simulink model "testSymbolDemodulator"  (R2024a)
settings: Solver=FixedStepDiscrete  StartTime=0.0  StopTime=20  RelTol=1e-3
undefined symbols (not defined in the file or in its folder): QAM
libraries: commdigbbndam3 x10, whdlmod x6, commdigbbndpm3 x2, dspsrcs4 x1
settings Model: DataTypeOverride=Off  Creator=cotti  LastModifiedBy=cotti
settings OptimizationCC: BlockReduction=off  ConditionallyExecuteInputs=off  DefaultParameterBehavior=Inlined  InheritOutputTypeSmallerThanSingle=on
settings DebuggingCC: ArtificialAlgebraicLoopMsg=error  SingleTaskRateTransMsg=error
settings HardwareCC: ProdBitPerPointer=32  ProdBitPerSizeT=32  ProdBitPerPtrDiffT=32  ProdLargestAtomicFloat=None  ProdIntDivRoundTo=Undefined  ProdEndianess=Unspecified  ProdWordSize=32  ProdHWDeviceType=ASIC/FPGA->ASIC/FPGA  TargetBitPerLong=64  TargetBitPerPointer=64  TargetBitPerSizeT=64  TargetBitPerPtrDiffT=64  TargetLongLongMode=on  TargetIntDivRoundTo=Zero  TargetEndianess=LittleEndian  TargetWordSize=64  TargetHWDeviceType=Custom Processor->MATLAB Host Computer  ProdEqTarget=off

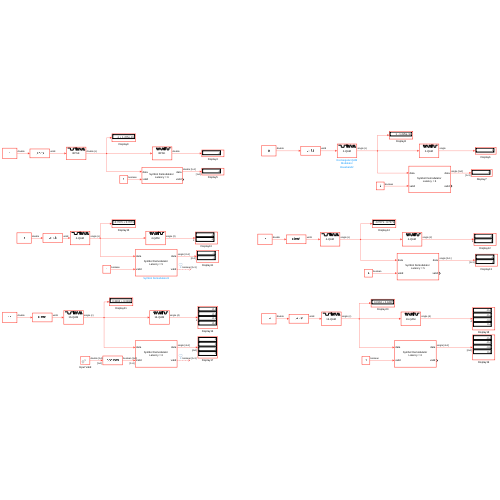
[thumbnail: Simulink's stored preview of the top-level diagram]
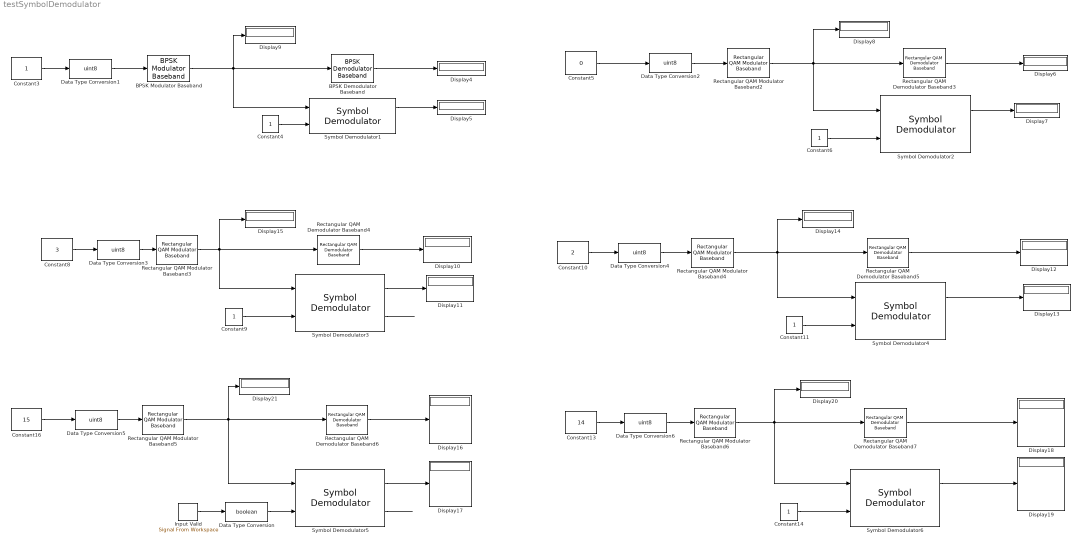
== system testSymbolDemodulator ==
  BPSK Demodulator Baseband : commdigbbndpm3/BPSK Demodulator Baseband  DecType=Approximate log-likelihood ratio  VarSource=Dialog  Variance=1  Ph=0  outDtype=Inherit via internal rule  derotateFactorWordLen=16  derotateFactorDataTypeStr=Inherit: Same word length as input  derotateFactorLastDataTypeStr=Inherit: Same word length as input
      settings: LibrarySourceBlock=|
      | commhdldigbbndpm/BPSK
      | Demodulator
      | Baseband
  BPSK Modulator Baseband : commdigbbndpm3/BPSK Modulator Baseband  Ph=0  outDtype=double  outWordLen=16  outUDDataType=sfix(16)  outFracLenMode=Best precision  outFracLen=15  outDataTypeStr=double  outLastDataTypeStr=double
      settings: LibrarySourceBlock=|
      | commhdldigbbndpm/BPSK
      | Modulator
      | Baseband
  Constant10 : Constant  Value=2  SampleTime=1
  Constant{4,6,9,11,14} (5 alike) : Constant  OutDataTypeStr=boolean  SampleTime=-1
  Constant13 : Constant  Value=14  SampleTime=1
  Constant16 : Constant  Value=15  SampleTime=1
  Constant3 : Constant  SampleTime=1
  Constant5 : Constant  Value=0  SampleTime=1
  Constant8 : Constant  Value=3  SampleTime=1
  Data Type Conversion : DataTypeConversion  OutDataTypeStr=boolean  SaturateOnIntegerOverflow=off  RndMeth=Floor
  Data Type Conversion{1..6} (6 alike) : DataTypeConversion  OutDataTypeStr=uint8  SaturateOnIntegerOverflow=off  RndMeth=Floor
  Display{4..21} (18 alike) : Display
  Input Valid : dspsrcs4/Signal From Workspace  X=1  Ts=1  nsamps=1  OutputAfterFinalValue=Setting to zero  ignoreOrWarnInputAndFrameLengths=off  OutputFrames=off
  Rectangular QAM Demodulator Baseband3 : commdigbbndam3/Rectangular QAM Demodulator Baseband  M=2  OutType=Bit  DecType=Approximate log-likelihood ratio  VarSource=Dialog  Variance=1  Dec=Binary  Mapping=[ 2, 3, 1, 0, 6, 7, 5, 4, 14, 15, 13, 12, 10, 11, 9, 8 ]  PowType=Average Power  MinDist=2  AvgPow=1  PeakPow=1  Ph=pi  outDtype1=Inherit via internal rule  outDtype2=Inherit via internal rule  derotateFactorWordLen=16  derotateFactorDataTypeStr=Inherit: Same word length as input  derotateFactorLastDataTypeStr=Inherit: Same word length as input  denormFactorWordLen=16  denormFactorDataTypeStr=Inherit: Same word length as input  denormFactorLastDataTypeStr=Inherit: Same word length as input  prodOutWordLen=32  prodOutOverflowMode=Wrap  prodOutRoundingMode=Floor  prodOutOvFlMode=off  prodOutOvFlModeLastStrValue=off  sumWordLen=32
      settings: LibrarySourceBlock=|
      | commhdldigbbndam/Rectangular QAM
      | Demodulator
      | Baseband
  Rectangular QAM Demodulator Baseband4 : commdigbbndam3/Rectangular QAM Demodulator Baseband  M=4  OutType=Bit  DecType=Approximate log-likelihood ratio  VarSource=Dialog  Variance=1  Dec=User-defined  Mapping=[3 2 1 0]  PowType=Average Power  MinDist=2  AvgPow=1  PeakPow=1  Ph=0  outDtype1=Inherit via internal rule  outDtype2=Inherit via internal rule  derotateFactorWordLen=16  derotateFactorDataTypeStr=Inherit: Same word length as input  derotateFactorLastDataTypeStr=Inherit: Same word length as input  denormFactorWordLen=16  denormFactorDataTypeStr=Inherit: Same word length as input  denormFactorLastDataTypeStr=Inherit: Same word length as input  prodOutWordLen=32  prodOutOverflowMode=Wrap  prodOutRoundingMode=Floor  prodOutOvFlMode=off  prodOutOvFlModeLastStrValue=off  sumWordLen=32
      settings: LibrarySourceBlock=|
      | commhdldigbbndam/Rectangular QAM
      | Demodulator
      | Baseband
  Rectangular QAM Demodulator Baseband5 : commdigbbndam3/Rectangular QAM Demodulator Baseband  M=4  OutType=Bit  DecType=Approximate log-likelihood ratio  VarSource=Dialog  Variance=1  Dec=User-defined  Mapping=qamTwoBits  PowType=Average Power  MinDist=2  AvgPow=1  PeakPow=1  Ph=0  outDtype1=Inherit via internal rule  outDtype2=Inherit via internal rule  derotateFactorWordLen=16  derotateFactorDataTypeStr=Inherit: Same word length as input  derotateFactorLastDataTypeStr=Inherit: Same word length as input  denormFactorWordLen=16  denormFactorDataTypeStr=Inherit: Same word length as input  denormFactorLastDataTypeStr=Inherit: Same word length as input  prodOutWordLen=32  prodOutOverflowMode=Wrap  prodOutRoundingMode=Floor  prodOutOvFlMode=off  prodOutOvFlModeLastStrValue=off  sumWordLen=32
      settings: LibrarySourceBlock=|
      | commhdldigbbndam/Rectangular QAM
      | Demodulator
      | Baseband
  Rectangular QAM Demodulator Baseband6 : commdigbbndam3/Rectangular QAM Demodulator Baseband  M=16  OutType=Bit  DecType=Approximate log-likelihood ratio  VarSource=Dialog  Variance=1  Dec=User-defined  Mapping=qamFourBits  PowType=Average Power  MinDist=2  AvgPow=1  PeakPow=1  Ph=0  outDtype1=Inherit via internal rule  outDtype2=Inherit via internal rule  derotateFactorWordLen=16  derotateFactorDataTypeStr=Inherit: Same word length as input  derotateFactorLastDataTypeStr=Inherit: Same word length as input  denormFactorWordLen=16  denormFactorDataTypeStr=Inherit: Same word length as input  denormFactorLastDataTypeStr=Inherit: Same word length as input  prodOutWordLen=32  prodOutOverflowMode=Wrap  prodOutRoundingMode=Floor  prodOutOvFlMode=off  prodOutOvFlModeLastStrValue=off  sumWordLen=32
      settings: LibrarySourceBlock=|
      | commhdldigbbndam/Rectangular QAM
      | Demodulator
      | Baseband
  Rectangular QAM Demodulator Baseband7 : commdigbbndam3/Rectangular QAM Demodulator Baseband  M=16  OutType=Bit  DecType=Approximate log-likelihood ratio  VarSource=Dialog  Variance=1  Dec=User-defined  Mapping=qamFourBits  PowType=Average Power  MinDist=2  AvgPow=1  PeakPow=1  Ph=0  outDtype1=Inherit via internal rule  outDtype2=Inherit via internal rule  derotateFactorWordLen=16  derotateFactorDataTypeStr=Inherit: Same word length as input  derotateFactorLastDataTypeStr=Inherit: Same word length as input  denormFactorWordLen=16  denormFactorDataTypeStr=Inherit: Same word length as input  denormFactorLastDataTypeStr=Inherit: Same word length as input  prodOutWordLen=32  prodOutOverflowMode=Wrap  prodOutRoundingMode=Floor  prodOutOvFlMode=off  prodOutOvFlModeLastStrValue=off  sumWordLen=32
      settings: LibrarySourceBlock=|
      | commhdldigbbndam/Rectangular QAM
      | Demodulator
      | Baseband
  Rectangular QAM Modulator Baseband2 : commdigbbndam3/Rectangular QAM Modulator Baseband  M=2  InType=Integer  Enc=Binary  Mapping=[0:15]  PowType=Average Power  MinDist=2  AvgPow=1  PeakPow=1  Ph=pi  outDtype=single  outWordLen=16  outUDDataType=sfix(16)  outFracLenMode=User-defined  outFracLen=14  outDataTypeStr=single  outLastDataTypeStr=single
      settings: LibrarySourceBlock=|
      | commhdldigbbndam/Rectangular QAM
      | Modulator
      | Baseband
  Rectangular QAM Modulator Baseband3 : commdigbbndam3/Rectangular QAM Modulator Baseband  M=4  InType=Integer  Enc=User-defined  Mapping=qamTwoBits  PowType=Average Power  MinDist=2  AvgPow=1  PeakPow=1  Ph=0  outDtype=single  outWordLen=16  outUDDataType=sfix(16)  outFracLenMode=User-defined  outFracLen=14  outDataTypeStr=single  outLastDataTypeStr=single
      settings: LibrarySourceBlock=|
      | commhdldigbbndam/Rectangular QAM
      | Modulator
      | Baseband
  Rectangular QAM Modulator Baseband4 : commdigbbndam3/Rectangular QAM Modulator Baseband  M=4  InType=Integer  Enc=User-defined  Mapping=qamTwoBits  PowType=Average Power  MinDist=2  AvgPow=1  PeakPow=1  Ph=0  outDtype=single  outWordLen=16  outUDDataType=sfix(16)  outFracLenMode=User-defined  outFracLen=14  outDataTypeStr=single  outLastDataTypeStr=single
      settings: LibrarySourceBlock=|
      | commhdldigbbndam/Rectangular QAM
      | Modulator
      | Baseband
  Rectangular QAM Modulator Baseband5 : commdigbbndam3/Rectangular QAM Modulator Baseband  M=16  InType=Integer  Enc=User-defined  Mapping=qamFourBits  PowType=Average Power  MinDist=2  AvgPow=1  PeakPow=1  Ph=0  outDtype=single  outWordLen=16  outUDDataType=sfix(16)  outFracLenMode=User-defined  outFracLen=14  outDataTypeStr=single  outLastDataTypeStr=single
      settings: LibrarySourceBlock=|
      | commhdldigbbndam/Rectangular QAM
      | Modulator
      | Baseband
  Rectangular QAM Modulator Baseband6 : commdigbbndam3/Rectangular QAM Modulator Baseband  M=16  InType=Integer  Enc=User-defined  Mapping=qamFourBits  PowType=Average Power  MinDist=2  AvgPow=1  PeakPow=1  Ph=0  outDtype=single  outWordLen=16  outUDDataType=sfix(16)  outFracLenMode=User-defined  outFracLen=14  outDataTypeStr=single  outLastDataTypeStr=single
      settings: LibrarySourceBlock=|
      | commhdldigbbndam/Rectangular QAM
      | Modulator
      | Baseband
  Symbol Demodulator1 : whdlmod/Symbol Demodulator  ModulationSource=Property  ModulationScheme=BPSK  MaxModulation=256-QAM  ConstOrder=Default  ConstMap=[ 2, 3, 1, 0, 6, 7, 5, 4, 14, 15, 13, 12, 10, 11, 9, 8 ]  DecisionType=Approximate log-likelihood ratio  PhaseOffset=0  OutputType=Vector  NormMethod=Unit average power  MinSymDistance=2  NoiseVariance=off  SimulateUsing=Code generation
  Symbol Demodulator2 : whdlmod/Symbol Demodulator  ModulationSource=Property  ModulationScheme=BPSK  MaxModulation=256-QAM  ConstOrder=Default  ConstMap=[ 2, 3, 1, 0, 6, 7, 5, 4, 14, 15, 13, 12, 10, 11, 9, 8 ]  DecisionType=Approximate log-likelihood ratio  PhaseOffset=0  OutputType=Vector  NormMethod=Unit average power  MinSymDistance=2  NoiseVariance=off  SimulateUsing=Code generation
  Symbol Demodulator3 : whdlmod/Symbol Demodulator  ModulationSource=Property  ModulationScheme=QPSK  MaxModulation=256-QAM  ConstOrder=Default  ConstMap=[ 2, 3, 1, 0, 6, 7, 5, 4, 14, 15, 13, 12, 10, 11, 9, 8 ]  DecisionType=Approximate log-likelihood ratio  PhaseOffset=-pi/4  OutputType=Vector  NormMethod=Unit average power  MinSymDistance=2  NoiseVariance=off  SimulateUsing=Code generation
  Symbol Demodulator4 : whdlmod/Symbol Demodulator  ModulationSource=Property  ModulationScheme=QPSK  MaxModulation=256-QAM  ConstOrder=Default  ConstMap=[ 2, 3, 1, 0, 6, 7, 5, 4, 14, 15, 13, 12, 10, 11, 9, 8 ]  DecisionType=Approximate log-likelihood ratio  PhaseOffset=-pi/4  OutputType=Vector  NormMethod=Unit average power  MinSymDistance=2  NoiseVariance=off  SimulateUsing=Code generation
  Symbol Demodulator5 : whdlmod/Symbol Demodulator  ModulationSource=Property  ModulationScheme=16-QAM  MaxModulation=256-QAM  ConstOrder=User-defined  ConstMap=qamFourBits  DecisionType=Approximate log-likelihood ratio  PhaseOffset=-pi/4  OutputType=Vector  NormMethod=Unit average power  MinSymDistance=2  NoiseVariance=off  SimulateUsing=Code generation
  Symbol Demodulator6 : whdlmod/Symbol Demodulator  ModulationSource=Property  ModulationScheme=16-QAM  MaxModulation=256-QAM  ConstOrder=User-defined  ConstMap=qamFourBits  DecisionType=Approximate log-likelihood ratio  PhaseOffset=-pi/4  OutputType=Vector  NormMethod=Unit average power  MinSymDistance=2  NoiseVariance=off  SimulateUsing=Code generation
  wires:
  Symbol Demodulator6/1 -> Display19/1
  Constant14/1 -> Symbol Demodulator6/2
  Constant10/1 -> Data Type Conversion4/1
  Constant11/1 -> Symbol Demodulator4/2
  Constant3/1 -> Data Type Conversion1/1
  Data Type Conversion5/1 -> Rectangular QAM Modulator Baseband5/1
  BPSK Demodulator Baseband/1 -> Display4/1
  Data Type Conversion1/1 -> BPSK Modulator Baseband/1
  Rectangular QAM Demodulator Baseband4/1 -> Display10/1
  Symbol Demodulator5/1 -> Display17/1
  Data Type Conversion3/1 -> Rectangular QAM Modulator Baseband3/1
  Constant13/1 -> Data Type Conversion6/1
  Symbol Demodulator1/1 -> Display5/1
  Constant5/1 -> Data Type Conversion2/1
  Rectangular QAM Demodulator Baseband5/1 -> Display12/1
  Constant8/1 -> Data Type Conversion3/1
  Data Type Conversion2/1 -> Rectangular QAM Modulator Baseband2/1
  Rectangular QAM Demodulator Baseband7/1 -> Display18/1
  Rectangular QAM Demodulator Baseband6/1 -> Display16/1
  Constant4/1 -> Symbol Demodulator1/2
  Rectangular QAM Modulator Baseband3/1 -> Display15/1, Symbol Demodulator3/1, Rectangular QAM Demodulator Baseband4/1
  Constant16/1 -> Data Type Conversion5/1
  Rectangular QAM Modulator Baseband4/1 -> Display14/1, Symbol Demodulator4/1, Rectangular QAM Demodulator Baseband5/1
  Data Type Conversion6/1 -> Rectangular QAM Modulator Baseband6/1
  Constant6/1 -> Symbol Demodulator2/2
  Symbol Demodulator3/1 -> Display11/1
  Rectangular QAM Demodulator Baseband3/1 -> Display6/1
  Constant9/1 -> Symbol Demodulator3/2
  Data Type Conversion4/1 -> Rectangular QAM Modulator Baseband4/1
  Rectangular QAM Modulator Baseband6/1 -> Display20/1, Symbol Demodulator6/1, Rectangular QAM Demodulator Baseband7/1
  Input Valid/1 -> Data Type Conversion/1
  Symbol Demodulator2/1 -> Display7/1
  Symbol Demodulator4/1 -> Display13/1
  Rectangular QAM Modulator Baseband5/1 -> Display21/1, Symbol Demodulator5/1, Rectangular QAM Demodulator Baseband6/1
  Rectangular QAM Modulator Baseband2/1 -> Display8/1, Symbol Demodulator2/1, Rectangular QAM Demodulator Baseband3/1
  BPSK Modulator Baseband/1 -> BPSK Demodulator Baseband/1, Display9/1, Symbol Demodulator1/1
  Symbol Demodulator5/2 -> ?
  Symbol Demodulator3/2 -> ?
  Data Type Conversion/1 -> Symbol Demodulator5/2
